simulink model "progetto"  (R2018b)
settings: Solver=VariableStepAuto  StartTime=0.0  StopTime=100  MaxStep=1e-3  RelTol=1e-3
settings Model: Creator=ACER-aspire  LastModifiedBy=ASUS
settings SFSimCC: SimUseLocalCustomCode=off
settings RTWCC: RTWUseLocalCustomCode=off

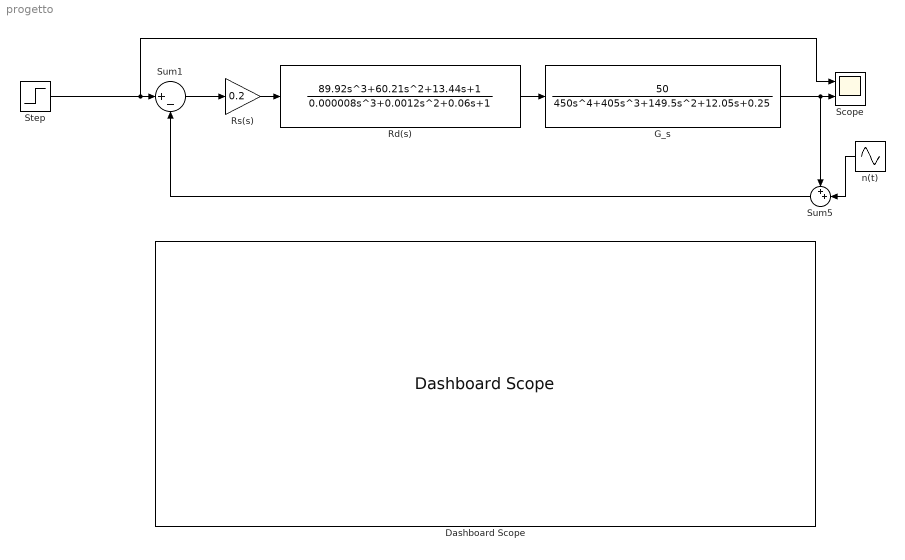
== system progetto ==
  Dashboard Scope : DashboardScope  WebBlockId=88  TimeSpan=80  Ymin=0  Ymax=1.2
  G_s : TransferFcn  Numerator=[50]  Denominator=[450 405 149.5 12.05 0.25]
  Rd(s) : TransferFcn  Numerator=[89.92 60.21 13.44 1]  Denominator=[0.000008 0.0012 0.06 1]
  Rs(s) : Gain  Gain=0.2
  Scope : Scope  NumInputPorts=2
  Step : Step  SampleTime=0
  Sum1 : Sum  Inputs=|+-
  Sum5 : Sum  Inputs=++|
  n(t) : Sin  Amplitude=0.015  Frequency=100  SampleTime=0
  wires:
  G_s/1 -> Scope/2, Sum5/1
  Sum5/1 -> Sum1/2
  Step/1 -> Sum1/1, Scope/1
  Sum1/1 -> Rs(s)/1
  n(t)/1 -> Sum5/2
  Rs(s)/1 -> Rd(s)/1
  Rd(s)/1 -> G_s/1
